simulink model "ParallelSimplified_inverter2201"  (R2022b)
settings: Solver=ode23t  StartTime=0.0  StopTime=5  MaxStep=1e-4  RelTol=1e-3
libraries: fl_lib x34, ee_lib x24, nesl_utility x9
settings Model: Creator=alexey  LastModifiedBy=alexey

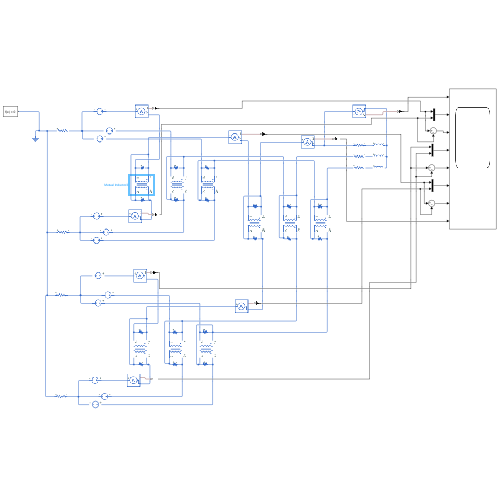
[thumbnail: Simulink's stored preview of the top-level diagram]
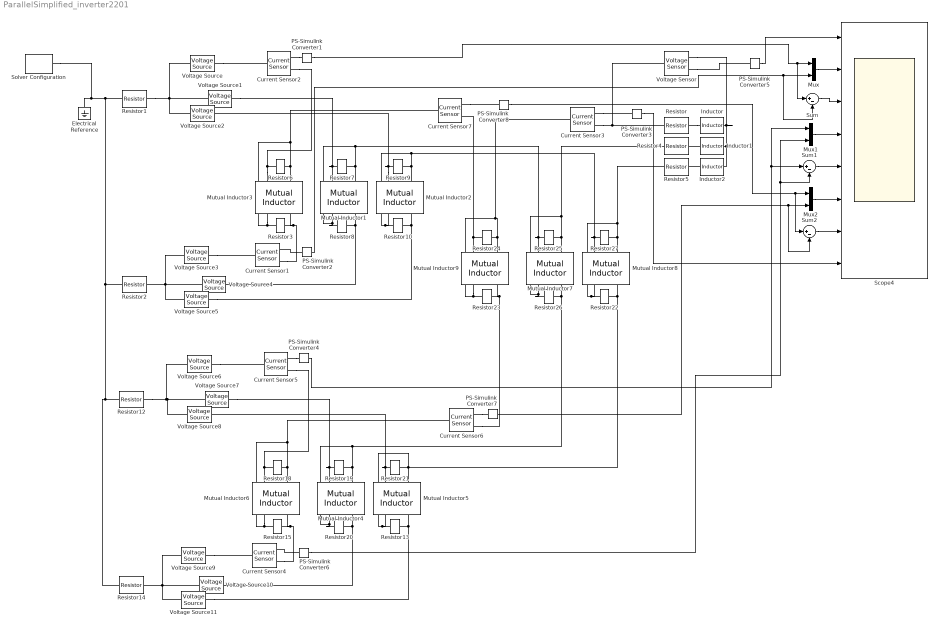
== system ParallelSimplified_inverter2201 ==
  Current Sensor{1..7} (7 alike) : fl_lib/Electrical/Electrical Sensors/Current Sensor
  Electrical Reference : fl_lib/Electrical/Electrical Elements/Electrical Reference
  Inductor : ee_lib/Passive/Inductor  l=3.8 mH  enable_L_tol=0  L_tol=20  tol_distribution=1  nSigma=4  r=0 Ohm  g=1e-9 1/Ohm  enable_operating_limits=0  operating_limit_action=2  max_working_current=1 A  power_rating=1 W  enable_faults=0  fault_action=1  lambdaPercent=50  k_faulted=0.9999  turnsShort=0  openCct=0  groundShort=0  groundShortG=0 1/Ohm  tau_fault=1e-3 s  enable_temporal_fault=0  t_fault=1 s  enable_behavioral_fault=0  max_permissible_voltage=100 V  n_fail_on_voltage=1  max_permissible_current=1 A  t_fail_on_current=1 s  i_L_specify=off  i_L_priority=High  i_L=0 A  i_L_nominal_specify=off  i_L_nominal_unit=A  i_L_nominal_value=1
  Inductor1 : ee_lib/Passive/Inductor  l=3.8 mH  enable_L_tol=0  L_tol=20  tol_distribution=1  nSigma=4  r=0 Ohm  g=1e-9 1/Ohm  enable_operating_limits=0  operating_limit_action=2  max_working_current=1 A  power_rating=1 W  enable_faults=0  fault_action=1  lambdaPercent=50  k_faulted=0.9999  turnsShort=0  openCct=0  groundShort=0  groundShortG=0 1/Ohm  tau_fault=1e-3 s  enable_temporal_fault=0  t_fault=1 s  enable_behavioral_fault=0  max_permissible_voltage=100 V  n_fail_on_voltage=1  max_permissible_current=1 A  t_fail_on_current=1 s  i_L_specify=off  i_L_priority=High  i_L=0 A  i_L_nominal_specify=off  i_L_nominal_unit=A  i_L_nominal_value=1
  Inductor2 : ee_lib/Passive/Inductor  l=3.8 mH  enable_L_tol=0  L_tol=20  tol_distribution=1  nSigma=4  r=0 Ohm  g=1e-9 1/Ohm  enable_operating_limits=0  operating_limit_action=2  max_working_current=1 A  power_rating=1 W  enable_faults=0  fault_action=1  lambdaPercent=50  k_faulted=0.9999  turnsShort=0  openCct=0  groundShort=0  groundShortG=0 1/Ohm  tau_fault=1e-3 s  enable_temporal_fault=0  t_fault=1 s  enable_behavioral_fault=0  max_permissible_voltage=100 V  n_fail_on_voltage=1  max_permissible_current=1 A  t_fail_on_current=1 s  i_L_specify=off  i_L_priority=High  i_L=0 A  i_L_nominal_specify=off  i_L_nominal_unit=A  i_L_nominal_value=1
  Mutual Inductor{1..9} (9 alike) : ee_lib/Passive/Transformers/Mutual Inductor  L1=500 uH  L2=500 uH  k=0.99999  L_tol=0  enable_L1_tol=0  L1_tol_distribution=1  L1_nSigma=4  enable_L2_tol=0  L2_tol_distribution=1  L2_nSigma=4  r=[4e-3, 4e-3] Ohm  g=[1e-03, 1e-03] 1/Ohm  enable_operating_limits=0  operating_limit_action=2  max_working_current=1 A  power_rating=1 W  enable_faults=simscape.enum.onoff.off  fault_action=simscape.enum.assert.action.none  fault_winding=1  lambdaPercent=50  turnsShort=ee.enum.faults.faultTurnsShort.no  openCct=ee.enum.faults.faultTurnsOpenCkt.no  groundShort=ee.enum.faults.faultTurnsGroundShort.no  groundShortG=0 1/Ohm  tau_fault=1e-3 s  enable_temporal_fault=ee.enum.faults.faultTriggerTemporal.no  t_fault=1 s  enable_behavioral_fault=ee.enum.faults.faultTriggerBehavioral.no  max_permissible_voltage=100 V  n_fail_on_voltage=1  max_permissible_current=1 A  t_fail_on_current=1 s  iL1_specify=off  iL1_priority=High  iL1=0 A  iL1_nominal_specify=off  iL1_nominal_unit=A  iL1_nominal_value=1  iL2_specify=off  iL2_priority=High  iL2=0 A  iL2_nominal_specify=off  iL2_nominal_unit=A  iL2_nominal_value=1
      settings: InternalSimscapePortConfiguration="{\"Bottom\":[],\"Left\":[{\"id\":\"p1\",\"label\":\"1+\",\"type\":\"foundation.electrical.electrical\"},{\"id\":\"n1\",\"label\":\"1-\",\"type\":\"foundation.electrical.electrical\"}],\"Right\":[{\"id\":\"p2\",\"label\":\"2+\",\"type\":\"foundation.electrical.electrical\"},{\"id\":\"n2\",\"label\":\"2-\",\"type\":\"foundation.electrical.electrical\"}],\"Top\":[]}"
  Mux : Mux  Inputs=2
  Mux1 : Mux  Inputs=2
  Mux2 : Mux  Inputs=2
  PS-Simulink Converter{1..8} (8 alike) : nesl_utility/PS-Simulink Converter  PhysicalDomain=network_engine_domain  SubClassName=ps_output  LeftPortType=input  RightPortType=output  PseudoPeriodic=off  Frequencies=[]  VectorFormat=1-D array  Unit=inherit  AffineConversion=off
  Resistor : fl_lib/Electrical/Electrical Elements/Resistor  R=2 Ohm  i_specify=off  i_priority=None  i=0 A  i_nominal_specify=off  i_nominal_unit=A  i_nominal_value=1  v_specify=off  v_priority=None  v=0 V  v_nominal_specify=off  v_nominal_unit=V  v_nominal_value=1
  Resistor{1..3,6..10,12..15,18..27} (22 alike) : fl_lib/Electrical/Electrical Elements/Resistor  R=1e6 Ohm  i_specify=off  i_priority=None  i=0 A  i_nominal_specify=off  i_nominal_unit=A  i_nominal_value=1  v_specify=off  v_priority=None  v=0 V  v_nominal_specify=off  v_nominal_unit=V  v_nominal_value=1
  Resistor4 : fl_lib/Electrical/Electrical Elements/Resistor  R=2 Ohm  i_specify=off  i_priority=None  i=0 A  i_nominal_specify=off  i_nominal_unit=A  i_nominal_value=1  v_specify=off  v_priority=None  v=0 V  v_nominal_specify=off  v_nominal_unit=V  v_nominal_value=1
  Resistor5 : fl_lib/Electrical/Electrical Elements/Resistor  R=2 Ohm  i_specify=off  i_priority=None  i=0 A  i_nominal_specify=off  i_nominal_unit=A  i_nominal_value=1  v_specify=off  v_priority=None  v=0 V  v_nominal_specify=off  v_nominal_unit=V  v_nominal_value=1
  Scope4 : Scope  NumInputPorts=8
  Solver Configuration : nesl_utility/Solver Configuration  PhysicalDomain=network_engine_domain  SubClassName=solver  LeftPortType=input  RightPortType=generic  Tones=[]  Harmonics=[]  SimulateNoise=off  Profile=off  UseLocalSampling=off  EnableSwitchedLinearOptims=on  FrequencyDomain=off  UseCCode=off  RelTol=0.001  AbsTol=0.001  MinStep=1e-09  ToWorkspace=off  RevertToSquareIcSolve=off  NumHomotopyIterations=100  PhasorMode=off  PhasorModeNumHarmonics=1  ConsistencySolver=NEWTON_XTOL_AFTER_FTOL  IndexReductionMethod=DerivativeReplacement  DoDC=off  ResidualTolerance=1e-09  ConsistencyTolSource=GLOBAL  ConsistencyAbsTol=0.001  ConsistencyRelTol=0.001  ConsistencyTolFactor=0.001  UseLocalSolver=off  LocalSolverChoice=NE_BACKWARD_EULER_ADVANCER  ResolveIndetEquations=on  FunctionEvalNumThread=1  LocalSolverSampleTime=0.001  DoFixedCost=off  MaxNonlinIter=3  MaxModeIter=2  ComputeImpulses=off  ImpulseIterations=2  LinearAlgebra=auto  LinearAlgebraNumThread=0  EquationFormulation=NE_TIME_EF  DelaysMemoryBudget=1024  AutomaticFiltering=on  FilteringTimeConstant=0.001  PartitionStorageMethod=AS_NEEDED  PartitionMemoryBudget=1024  PartitionMethod=ROBUST
  Sum : Sum  Inputs=|+-
  Sum1 : Sum  Inputs=|+-
  Sum2 : Sum  Inputs=|+-
  Voltage Sensor : fl_lib/Electrical/Electrical Sensors/Voltage Sensor
  Voltage Source : ee_lib/Sources/Voltage Source  dc_voltage=0 V  ac_voltage=311 V  ac_shift=0 deg  ac_frequency=50 Hz  noise_mode=ee.enum.sources.noise.Disabled  PSD=0 V^2/Hz  sample_time=1e-3 s  repeatability=ee.enum.sources.repeatability.NotRepeatable  user_seed=0  auto_seed=3499211588  i_specify=off  i_priority=None  i=0 A  i_nominal_specify=off  i_nominal_unit=A  i_nominal_value=1  v_specify=off  v_priority=None  v=0 V  v_nominal_specify=off  v_nominal_unit=V  v_nominal_value=1
  Voltage Source1 : ee_lib/Sources/Voltage Source  dc_voltage=0 V  ac_voltage=311 V  ac_shift=120 deg  ac_frequency=50 Hz  noise_mode=ee.enum.sources.noise.Disabled  PSD=0 V^2/Hz  sample_time=1e-3 s  repeatability=ee.enum.sources.repeatability.NotRepeatable  user_seed=0  auto_seed=3890346746  i_specify=off  i_priority=None  i=0 A  i_nominal_specify=off  i_nominal_unit=A  i_nominal_value=1  v_specify=off  v_priority=None  v=0 V  v_nominal_specify=off  v_nominal_unit=V  v_nominal_value=1
  Voltage Source10 : ee_lib/Sources/Voltage Source  dc_voltage=0 V  ac_voltage=310 V  ac_shift=120.1 deg  ac_frequency=50 Hz  noise_mode=ee.enum.sources.noise.Disabled  PSD=0 V^2/Hz  sample_time=1e-3 s  repeatability=ee.enum.sources.repeatability.NotRepeatable  user_seed=0  auto_seed=1811450916  i_specify=off  i_priority=None  i=0 A  i_nominal_specify=off  i_nominal_unit=A  i_nominal_value=1  v_specify=off  v_priority=None  v=0 V  v_nominal_specify=off  v_nominal_unit=V  v_nominal_value=1
  Voltage Source11 : ee_lib/Sources/Voltage Source  dc_voltage=0 V  ac_voltage=310 V  ac_shift=240.1 deg  ac_frequency=50 Hz  noise_mode=ee.enum.sources.noise.Disabled  PSD=0 V^2/Hz  sample_time=1e-3 s  repeatability=ee.enum.sources.repeatability.NotRepeatable  user_seed=0  auto_seed=3933054132  i_specify=off  i_priority=None  i=0 A  i_nominal_specify=off  i_nominal_unit=A  i_nominal_value=1  v_specify=off  v_priority=None  v=0 V  v_nominal_specify=off  v_nominal_unit=V  v_nominal_value=1
  Voltage Source2 : ee_lib/Sources/Voltage Source  dc_voltage=0 V  ac_voltage=311 V  ac_shift=240 deg  ac_frequency=50 Hz  noise_mode=ee.enum.sources.noise.Disabled  PSD=0 V^2/Hz  sample_time=1e-3 s  repeatability=ee.enum.sources.repeatability.NotRepeatable  user_seed=0  auto_seed=545404223  i_specify=off  i_priority=None  i=0 A  i_nominal_specify=off  i_nominal_unit=A  i_nominal_value=1  v_specify=off  v_priority=None  v=0 V  v_nominal_specify=off  v_nominal_unit=V  v_nominal_value=1
  Voltage Source3 : ee_lib/Sources/Voltage Source  dc_voltage=0 V  ac_voltage=311 V  ac_shift=0.1 deg  ac_frequency=50 Hz  noise_mode=ee.enum.sources.noise.Disabled  PSD=0 V^2/Hz  sample_time=1e-3 s  repeatability=ee.enum.sources.repeatability.NotRepeatable  user_seed=0  auto_seed=2084672538  i_specify=off  i_priority=None  i=0 A  i_nominal_specify=off  i_nominal_unit=A  i_nominal_value=1  v_specify=off  v_priority=None  v=0 V  v_nominal_specify=off  v_nominal_unit=V  v_nominal_value=1
  Voltage Source4 : ee_lib/Sources/Voltage Source  dc_voltage=0 V  ac_voltage=311 V  ac_shift=120.1 deg  ac_frequency=50 Hz  noise_mode=ee.enum.sources.noise.Disabled  PSD=0 V^2/Hz  sample_time=1e-3 s  repeatability=ee.enum.sources.repeatability.NotRepeatable  user_seed=0  auto_seed=3437178441  i_specify=off  i_priority=None  i=0 A  i_nominal_specify=off  i_nominal_unit=A  i_nominal_value=1  v_specify=off  v_priority=None  v=0 V  v_nominal_specify=off  v_nominal_unit=V  v_nominal_value=1
  Voltage Source5 : ee_lib/Sources/Voltage Source  dc_voltage=0 V  ac_voltage=311 V  ac_shift=240.1 deg  ac_frequency=50 Hz  noise_mode=ee.enum.sources.noise.Disabled  PSD=0 V^2/Hz  sample_time=1e-3 s  repeatability=ee.enum.sources.repeatability.NotRepeatable  user_seed=0  auto_seed=609397185  i_specify=off  i_priority=None  i=0 A  i_nominal_specify=off  i_nominal_unit=A  i_nominal_value=1  v_specify=off  v_priority=None  v=0 V  v_nominal_specify=off  v_nominal_unit=V  v_nominal_value=1
  Voltage Source6 : ee_lib/Sources/Voltage Source  dc_voltage=0 V  ac_voltage=312 V  ac_shift=0 deg  ac_frequency=50 Hz  noise_mode=ee.enum.sources.noise.Disabled  PSD=0 V^2/Hz  sample_time=1e-3 s  repeatability=ee.enum.sources.repeatability.NotRepeatable  user_seed=0  auto_seed=3402504572  i_specify=off  i_priority=None  i=0 A  i_nominal_specify=off  i_nominal_unit=A  i_nominal_value=1  v_specify=off  v_priority=None  v=0 V  v_nominal_specify=off  v_nominal_unit=V  v_nominal_value=1
  Voltage Source7 : ee_lib/Sources/Voltage Source  dc_voltage=0 V  ac_voltage=312 V  ac_shift=120 deg  ac_frequency=50 Hz  noise_mode=ee.enum.sources.noise.Disabled  PSD=0 V^2/Hz  sample_time=1e-3 s  repeatability=ee.enum.sources.repeatability.NotRepeatable  user_seed=0  auto_seed=4120988592  i_specify=off  i_priority=None  i=0 A  i_nominal_specify=off  i_nominal_unit=A  i_nominal_value=1  v_specify=off  v_priority=None  v=0 V  v_nominal_specify=off  v_nominal_unit=V  v_nominal_value=1
  Voltage Source8 : ee_lib/Sources/Voltage Source  dc_voltage=0 V  ac_voltage=312 V  ac_shift=240 deg  ac_frequency=50 Hz  noise_mode=ee.enum.sources.noise.Disabled  PSD=0 V^2/Hz  sample_time=1e-3 s  repeatability=ee.enum.sources.repeatability.NotRepeatable  user_seed=0  auto_seed=2816384857  i_specify=off  i_priority=None  i=0 A  i_nominal_specify=off  i_nominal_unit=A  i_nominal_value=1  v_specify=off  v_priority=None  v=0 V  v_nominal_specify=off  v_nominal_unit=V  v_nominal_value=1
  Voltage Source9 : ee_lib/Sources/Voltage Source  dc_voltage=0 V  ac_voltage=310 V  ac_shift=0.1 deg  ac_frequency=50 Hz  noise_mode=ee.enum.sources.noise.Disabled  PSD=0 V^2/Hz  sample_time=1e-3 s  repeatability=ee.enum.sources.repeatability.NotRepeatable  user_seed=0  auto_seed=153380492  i_specify=off  i_priority=None  i=0 A  i_nominal_specify=off  i_nominal_unit=A  i_nominal_value=1  v_specify=off  v_priority=None  v=0 V  v_nominal_specify=off  v_nominal_unit=V  v_nominal_value=1
  wires:
  PS-Simulink Converter5/1 -> Scope4/1
  PS-Simulink Converter1/1 -> Sum/1, Mux/1
  PS-Simulink Converter2/1 -> Sum/2, Mux/2
  PS-Simulink Converter8/1 -> Sum2/1, Mux2/1
  Mux/1 -> Scope4/2
  Sum/1 -> Scope4/3
  Sum1/1 -> Scope4/5
  Mux1/1 -> Scope4/4
  PS-Simulink Converter7/1 -> Sum2/2, Mux2/2
  PS-Simulink Converter6/1 -> Mux1/2, Sum1/2
  PS-Simulink Converter4/1 -> Sum1/1, Mux1/1
  Mux2/1 -> Scope4/6
  Sum2/1 -> Scope4/7
  PS-Simulink Converter3/1 -> Scope4/8
  connections:
  Voltage Sensor/RConn2 -- Inductor/RConn1 -- Inductor1/RConn1 -- Inductor2/RConn1
  Voltage Sensor/RConn1 -- PS-Simulink Converter5/LConn1
  Voltage Source2/RConn1 -- Voltage Source/RConn1 -- Resistor1/RConn1 -- Voltage Source1/RConn1
  Resistor14/LConn1 -- Resistor1/LConn1 -- Solver Configuration/RConn1 -- Electrical Reference/LConn1 -- Resistor2/LConn1 -- Resistor12/LConn1
  Voltage Source3/RConn1 -- Voltage Source5/RConn1 -- Voltage Source4/RConn1 -- Resistor2/RConn1
  Mutual Inductor3/LConn2 -- Current Sensor2/RConn2 -- Resistor6/LConn1
  Resistor3/RConn1 -- Current Sensor1/RConn2 -- Mutual Inductor3/RConn1
  Mutual Inductor1/RConn1 -- Voltage Source4/LConn1 -- Resistor8/RConn1
  Mutual Inductor2/RConn1 -- Voltage Source5/LConn1 -- Resistor10/RConn1
  Voltage Sensor/LConn1 -- Current Sensor3/RConn2 -- Resistor/LConn1
  Resistor27/LConn1 -- Resistor10/LConn1 -- Mutual Inductor2/RConn2 -- Resistor9/RConn1 -- Mutual Inductor2/LConn1 -- Mutual Inductor8/LConn2
  Voltage Source3/LConn1 -- Current Sensor1/LConn1
  PS-Simulink Converter2/LConn1 -- Current Sensor1/RConn1
  Current Sensor2/RConn1 -- PS-Simulink Converter1/LConn1
  Current Sensor3/RConn1 -- PS-Simulink Converter3/LConn1
  Resistor/RConn1 -- Inductor/LConn1
  Inductor1/LConn1 -- Resistor4/RConn1
  Inductor2/LConn1 -- Resistor5/RConn1
  Voltage Source/LConn1 -- Current Sensor2/LConn1
  Resistor7/LConn1 -- Voltage Source1/LConn1 -- Mutual Inductor1/LConn2
  Mutual Inductor2/LConn2 -- Voltage Source2/LConn1 -- Resistor9/LConn1
  Voltage Source6/RConn1 -- Resistor12/RConn1 -- Voltage Source8/RConn1 -- Voltage Source7/RConn1
  Voltage Source11/RConn1 -- Resistor14/RConn1 -- Voltage Source10/RConn1 -- Voltage Source9/RConn1
  Current Sensor5/RConn2 -- Mutual Inductor6/LConn2 -- Resistor18/LConn1
  Current Sensor4/RConn2 -- Mutual Inductor6/RConn1 -- Resistor15/RConn1
  Voltage Source10/LConn1 -- Mutual Inductor4/RConn1 -- Resistor20/RConn1
  Voltage Source11/LConn1 -- Mutual Inductor5/RConn1 -- Resistor13/RConn1
  Mutual Inductor6/LConn1 -- Resistor18/RConn1 -- Current Sensor6/LConn1 -- Resistor15/LConn1 -- Mutual Inductor6/RConn2
  Voltage Source7/LConn1 -- Mutual Inductor4/LConn2 -- Resistor19/LConn1
  Voltage Source8/LConn1 -- Mutual Inductor5/LConn2 -- Resistor21/LConn1
  Voltage Source9/LConn1 -- Current Sensor4/LConn1
  PS-Simulink Converter6/LConn1 -- Current Sensor4/RConn1
  Current Sensor5/RConn1 -- PS-Simulink Converter4/LConn1
  Current Sensor6/RConn1 -- PS-Simulink Converter7/LConn1
  Voltage Source6/LConn1 -- Current Sensor5/LConn1
  Mutual Inductor3/RConn2 -- Mutual Inductor3/LConn1 -- Resistor6/RConn1 -- Current Sensor7/LConn1 -- Resistor3/LConn1
  Resistor23/RConn1 -- Current Sensor6/RConn2 -- Mutual Inductor9/RConn1
  Resistor20/LConn1 -- Mutual Inductor4/RConn2 -- Mutual Inductor7/RConn1 -- Resistor26/RConn1 -- Mutual Inductor4/LConn1 -- Resistor19/RConn1
  Resistor13/LConn1 -- Mutual Inductor5/RConn2 -- Mutual Inductor8/RConn1 -- Resistor22/RConn1 -- Mutual Inductor5/LConn1 -- Resistor21/RConn1
  Resistor22/LConn1 -- Mutual Inductor8/RConn2 -- Mutual Inductor8/LConn1 -- Resistor27/RConn1 -- Resistor5/LConn1
  Resistor26/LConn1 -- Mutual Inductor7/RConn2 -- Mutual Inductor7/LConn1 -- Resistor25/RConn1 -- Resistor4/LConn1
  Mutual Inductor9/LConn1 -- Resistor24/RConn1 -- Current Sensor3/LConn1 -- Resistor23/LConn1 -- Mutual Inductor9/RConn2
  Resistor8/LConn1 -- Mutual Inductor7/LConn2 -- Resistor25/LConn1 -- Resistor7/RConn1 -- Mutual Inductor1/LConn1 -- Mutual Inductor1/RConn2
  Current Sensor7/RConn1 -- PS-Simulink Converter8/LConn1
  Resistor24/LConn1 -- Current Sensor7/RConn2 -- Mutual Inductor9/LConn2
